simulink model "fINAL_SIMULINK"  (R2023a)
settings: Solver=VariableStepAuto  StartTime=0.0  StopTime=60  RelTol=1e-3
undefined symbols (not defined in the file): A, B, C, D, K
libraries: simulink_extras x2
settings Model: Creator=nm.gomeza1  LastModifiedBy=nm.gomeza1

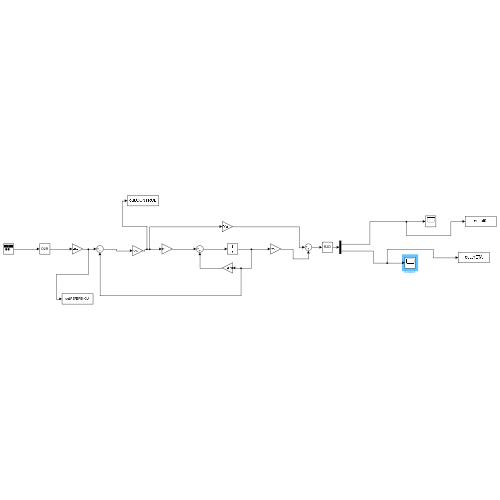
[thumbnail: Simulink's stored preview of the top-level diagram]
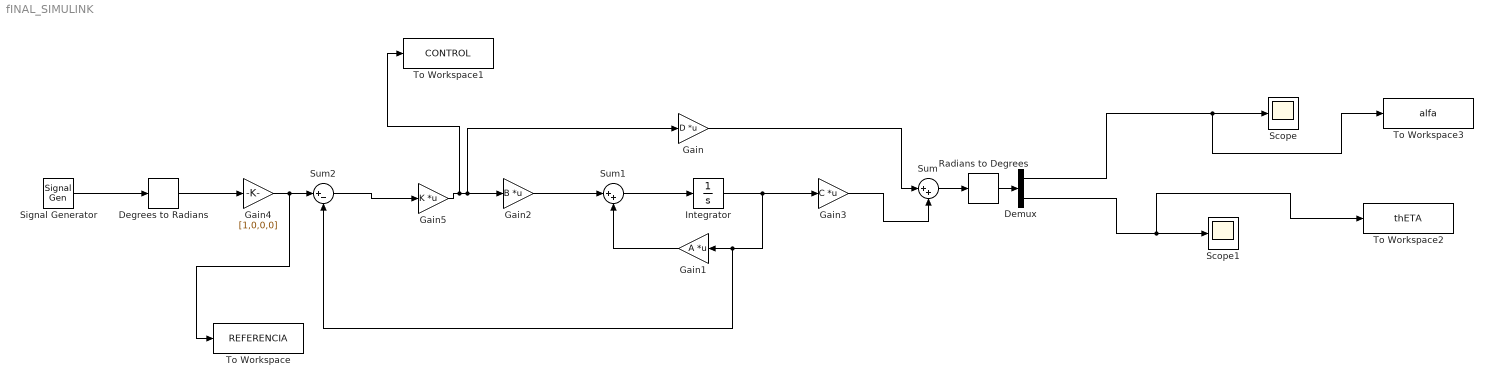
== system fINAL_SIMULINK ==
  Degrees to Radians : simulink_extras/Transformations/Degrees to Radians
  Demux : Demux  Outputs=2
  Gain : Gain  Gain=D  Multiplication=Matrix(K*u)
  Gain1 : Gain  Gain=A  Multiplication=Matrix(K*u)
  Gain2 : Gain  Gain=B  Multiplication=Matrix(K*u)
  Gain3 : Gain  Gain=C  Multiplication=Matrix(K*u)
  Gain4 : Gain  Gain=[1,0,0,0]
  Gain5 : Gain  Gain=K  Multiplication=Matrix(K*u)
  Integrator : Integrator
  Radians to Degrees : simulink_extras/Transformations/Radians to Degrees
  Scope : Scope
  Scope1 : Scope
  Signal Generator : SignalGenerator  WaveForm=square  Amplitude=20  Frequency=0.1
  Sum : Sum  Inputs=|++
  Sum1 : Sum  Inputs=|++
  Sum2 : Sum  Inputs=|+-
  To Workspace : ToWorkspace  VariableName=REFERENCIA  SaveFormat=Timeseries  SampleTime=-1
  To Workspace1 : ToWorkspace  VariableName=CONTROL  SaveFormat=Timeseries  SampleTime=-1
  To Workspace2 : ToWorkspace  VariableName=thETA  SaveFormat=Timeseries  SampleTime=-1
  To Workspace3 : ToWorkspace  VariableName=alfa  SaveFormat=Timeseries  SampleTime=-1
  wires:
  Gain2/1 -> Sum1/1
  Sum1/1 -> Integrator/1
  Integrator/1 -> Sum2/2, Gain1/1, Gain3/1
  Gain3/1 -> Sum/2
  Gain/1 -> Sum/1
  Gain1/1 -> Sum1/2
  Signal Generator/1 -> Degrees to Radians/1
  Degrees to Radians/1 -> Gain4/1
  Gain4/1 -> To Workspace/1, Sum2/1
  Gain5/1 -> To Workspace1/1, Gain/1, Gain2/1
  Sum2/1 -> Gain5/1
  Sum/1 -> Radians to Degrees/1
  Radians to Degrees/1 -> Demux/1
  Demux/1 -> To Workspace3/1, Scope/1
  Demux/2 -> To Workspace2/1, Scope1/1
